simulink model "WithoutIsNew"  (R2017a)
settings: Solver=FixedStepAuto  StartTime=0.0  StopTime=10.0  FixedStep=0.01  RelTol=1e-3
undefined symbols (not defined in the file): Point
libraries: robotlib x3
settings Model: Creator=marco  LastModifiedBy=marco
settings OptimizationCC: PassReuseOutputArgsAs=Individual arguments  MaxStackSize=64
settings DebuggingCC: ParameterTunabilityLossMsg=error
settings HardwareCC: ProdBitPerPointer=32  ProdBitPerSizeT=32  ProdBitPerPtrDiffT=32  ProdLargestAtomicFloat=None  ProdIntDivRoundTo=Undefined  ProdEndianess=Unspecified  ProdWordSize=32  ProdHWDeviceType=Generic->Unspecified (assume 32-bit Generic)
settings SFSimCC: MATLABDynamicMemAlloc=off
settings RTWCC: SystemTargetFile=ert.tlc  HardwareBoard=Robot Operating System (ROS)  TLCOptions="-aInlineSetEventsForThisBaseRateFcn=TLC_FALSE -aSuppressMultiTaskScheduler=TLC_FALSE  -aRateBasedStepFcn=0"  TemplateMakefile=ert_default_tmf  Description=Embedded Coder  GenerateReport=on  Toolchain=Catkin  IncludeHyperlinkInReport=on  LaunchReport=on  TargetLang=C++  GenerateTraceInfo=on  GenerateTraceReport=on  GenerateTraceReportSl=on  GenerateTraceReportSf=on  GenerateTraceReportEml=on
settings CodeAppCC: ForceParamTrailComments=on  IgnoreCustomStorageClasses=off  OperatorAnnotations=on  SimulinkDataObjDesc=on  SFDataObjDesc=on  MATLABFcnDesc=on  InsertBlockDesc=on  MATLABSourceComments=on
settings ERTTargetCC: SupportContinuousTime=on

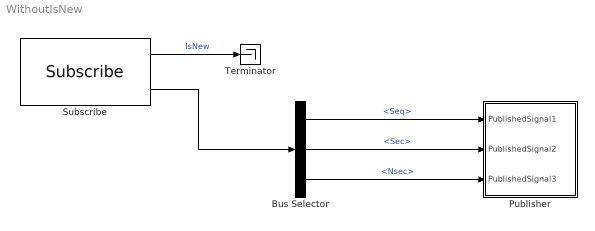
== system WithoutIsNew ==
  Bus Selector : BusSelector  OutputSignals=Header.Seq,Header.Stamp.Sec,Header.Stamp.Nsec
  Publisher : Subsystem
  Subscribe : robotlib/Subscribe  SourceLibraryInfo=This block requires Robotics System Toolbox  topicSource=Specify your own  topic=/chatter  messageType=geometry_msgs/PoseArray  sampleTime=-1  messageQueueLength=1
      settings: SourceProductBaseCode=RO
  Terminator : Terminator
  wires:
  Subscribe/2 -> Bus Selector/1
  Bus Selector/1 -> Publisher/1(PublishedSignal1)  "<Seq>"
  Bus Selector/2 -> Publisher/2(PublishedSignal2)  "<Sec>"
  Bus Selector/3 -> Publisher/3(PublishedSignal3)  "<Nsec>"
  Subscribe/1 -> Terminator/1  "IsNew"

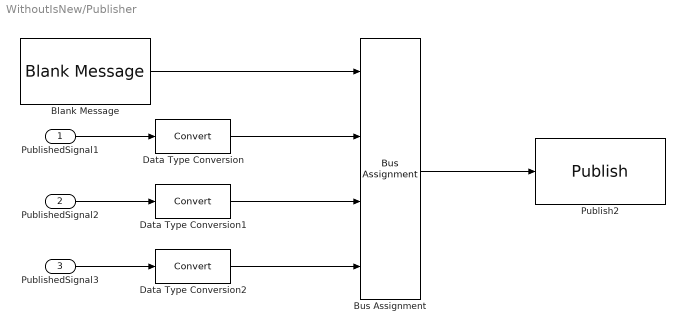
== system WithoutIsNew/Publisher ==
  PublishedSignal1 : Inport
  PublishedSignal2 : Inport  Port=2
  PublishedSignal3 : Inport  Port=3
  Blank Message : robotlib/Blank Message  SourceLibraryInfo=This block requires Robotics System Toolbox  messageType=geometry_msgs/PointStamped  SampleTime=inf
      settings: SourceProductBaseCode=RO
  Bus Assignment : BusAssignment  AssignedSignals=Point.X,Point.Y,Point.Z
  Data Type Conversion : DataTypeConversion
  Data Type Conversion1 : DataTypeConversion
  Data Type Conversion2 : DataTypeConversion
  Publish2 : robotlib/Publish  SourceLibraryInfo=This block requires Robotics System Toolbox  topicSource=Specify your own  topic=/Chatter_WithoutIsNew  messageType=geometry_msgs/PointStamped  messageQueueLength=1
      settings: SourceProductBaseCode=RO
  wires:
  PublishedSignal2/1 -> Data Type Conversion1/1
  Data Type Conversion/1 -> Bus Assignment/2
  Data Type Conversion1/1 -> Bus Assignment/3
  Bus Assignment/1 -> Publish2/1
  PublishedSignal3/1 -> Data Type Conversion2/1
  Data Type Conversion2/1 -> Bus Assignment/4
  PublishedSignal1/1 -> Data Type Conversion/1
  Blank Message/1 -> Bus Assignment/1
